simulink model "FIR"  (R2020b)
settings: Solver=VariableStepAuto  StartTime=0.0  StopTime=10.0  RelTol=1e-3
libraries: simulink x1
settings Model: Creator=Akshata Ashok  LastModifiedBy=Akshata Ashok

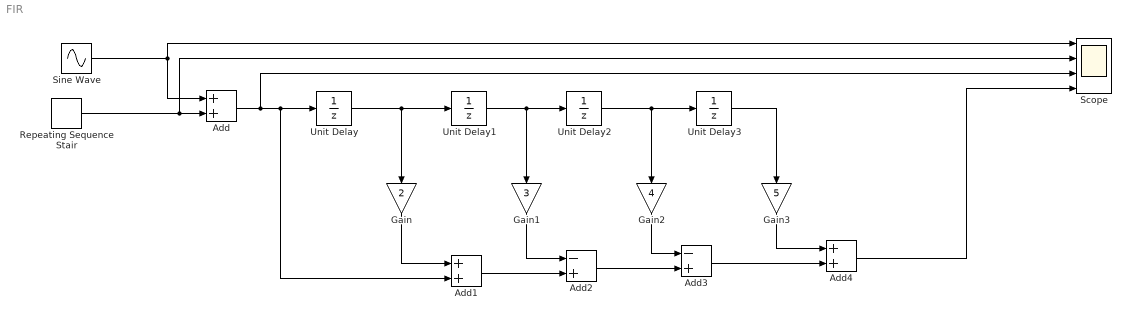
== system FIR ==
  Add : Sum
  Add1 : Sum
  Add2 : Sum  Inputs=-+
  Add3 : Sum  Inputs=-+
  Add4 : Sum
  Gain : Gain  Gain=2
  Gain1 : Gain  Gain=3
  Gain2 : Gain  Gain=4
  Gain3 : Gain  Gain=5
  Repeating Sequence Stair : simulink/Sources/Repeating Sequence Stair  OutValues=[3 1 4 2 1].'  tsamp=-1  OutMin=[]  OutMax=[]  OutDataTypeStr=double  OutputDataTypeScalingMode=double  OutDataType=fixdt(0,8)  ConRadixGroup=Best Precision: Vector-wise  OutScaling=2^-12
  Scope : Scope  NumInputPorts=4
  Sine Wave : Sin  Frequency=10  SampleTime=0
  Unit Delay{,1..3} (4 alike) : UnitDelay  SampleTime=-1  HasFrameUpgradeWarning=on
  wires:
  Sine Wave/1 -> Add/1, Scope/1
  Repeating Sequence Stair/1 -> Scope/2, Add/2
  Unit Delay/1 -> Gain/1, Unit Delay1/1
  Unit Delay1/1 -> Gain1/1, Unit Delay2/1
  Unit Delay2/1 -> Gain2/1, Unit Delay3/1
  Add/1 -> Scope/3, Add1/2, Unit Delay/1
  Unit Delay3/1 -> Gain3/1
  Gain/1 -> Add1/1
  Gain1/1 -> Add2/1
  Add1/1 -> Add2/2
  Gain2/1 -> Add3/1
  Add2/1 -> Add3/2
  Gain3/1 -> Add4/1
  Add3/1 -> Add4/2
  Add4/1 -> Scope/4
